simulink model "bus_as_currsource_charging_discharging_final_rearranged"  (R2023a)
settings: Solver=VariableStepAuto  StartTime=0.0  StopTime=10.0  RelTol=1e-3
libraries: spsParallelRLCBranchLib x72, spsCurrentMeasurementLib x27, spsVoltageMeasurementLib x27, spspowerguiLib x25, spsControlledVoltageSourceLib x24, spsVariableResistorLib x24, spsSeriesRLCBranchLib x6, spsMosfetLib x2, sdolib x1, spsControlledCurrentSourceLib x1, spsGroundLib x1
(part 2 of 4)

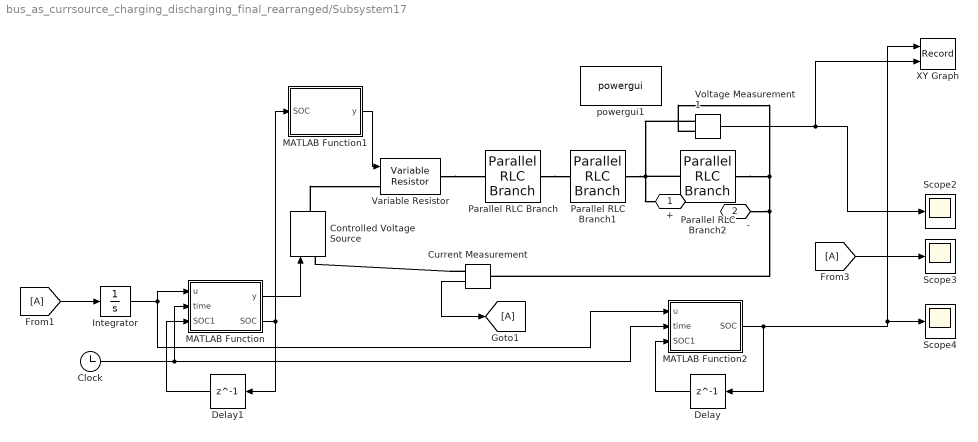
== system bus_as_currsource_charging_discharging_final_rearranged/Subsystem17 ==
  Clock : Clock
  Controlled Voltage Source : spsControlledVoltageSourceLib/Controlled Voltage Source  Initialize=on  Source_Type=DC  Amplitude=0  Phase=0  Frequency=0  Measurements=None
  Current Measurement : spsCurrentMeasurementLib/Current Measurement  PhasorSimulation=off  OutputType=Complex  PSBequivalent=0
  Delay : Delay  DelayLength=1  InitialCondition=0
  Delay1 : Delay  DelayLength=1  InitialCondition=0
  From1 : From
  From3 : From
  Goto1 : Goto
  Integrator : Integrator
  MATLAB Function : MATLAB Function  TreatAsAtomicUnit=on
  MATLAB Function1 : MATLAB Function  TreatAsAtomicUnit=on
  MATLAB Function2 : MATLAB Function  TreatAsAtomicUnit=on
  Parallel RLC Branch : spsParallelRLCBranchLib/Parallel RLC Branch  LConnTagsString=a  RConnTagsString=__new0  BranchType=RC  Resistance=15.5e-3  Inductance=1e-3  SetiL0=off  InitialCurrent=0  Capacitance=1028.7  Setx0=off  InitialVoltage=0  Measurements=None
  Parallel RLC Branch1 : spsParallelRLCBranchLib/Parallel RLC Branch  LConnTagsString=a  RConnTagsString=__new0  BranchType=RC  Resistance=18.3e-3  Inductance=1e-3  SetiL0=off  InitialCurrent=0  Capacitance=5756.6  Setx0=off  InitialVoltage=0  Measurements=None
  Parallel RLC Branch2 : spsParallelRLCBranchLib/Parallel RLC Branch  LConnTagsString=a  RConnTagsString=__new0  BranchType=R  Resistance=1e9  Inductance=1e-3  SetiL0=off  InitialCurrent=0  Capacitance=5756.6  Setx0=off  InitialVoltage=0  Measurements=None
  Scope2 : Scope
  Scope3 : Scope
  Scope4 : Scope
  Variable Resistor : spsVariableResistorLib/Variable Resistor  Rabsmin=1e-3
      settings: LibrarySourceBlock=sps_lib/Passives/Variable Resistor
  Voltage Measurement1 : spsVoltageMeasurementLib/Voltage Measurement  PhasorSimulation=off  OutputType=Complex  PSBequivalent=0
  XY Graph : Record  FileSettingsInternal="{\"entries\":[{\"content\":{\"excelSettings\":{\"content\":{},\"type\":\"Streamout.ExcelSettings\"}},\"type\":\"Streamout.FileSettingStorage\",\"uuid\":\"ba5f6825-ae84-49c8-9f06-d48f38ab3e7c\"}],\"packageUris\":[\"http://schema.mathworks.com/mf0/streamout_blocks/R2020a\"],\"version\":\"1.0\"}"  Layout=[1 1]  SignalsInternal="{\"entries\":[{\"content\":{\"signals\":[{\"content\":{\"blockPath\":[\"untitled/Subsystem17/XY Graph\"],\"dimensions\":[1],\"domain\":\"untitled/Subsystem17/XY Graph\",\"lineColor\":\"#ff6929\",\"port\":1,\"signalID\":782,\"signalName\":\"MATLAB Function2\"},\"type\":\"RecordBlkView.Signal\",\"uuid\":\"a10a1c50-d255-4169-acf7-794a73575721\"},{\"content\":{\"blockPath\":[\"untitled/Subsystem17/XY Graph\"],\"dimensions\":[1],\"domain\":\"untitled/Subsystem17/XY Graph\",\"lineColor\":\"#b746ff\",\"port\":2,\"signalID\":785,\"signalName\":\"Voltage Measurement1\"},\"type\":\"RecordBlkView.Signal\",\"uuid\":\"1a7b2192-97ab-4747-8306-6a319dd4fa57\"}]},\"type\":\"RecordBlkView.InputSignals\",\"uuid\":\"436618d9-ba51-4f23-94da-7eccc7c92e1d\"}],\"packageUris\":[\"http://schema.mathworks.com/mf0/streamout_blocks/R2020a\"],\"version\":\"1.0\"}"  VisualizationBindings="{\"xyplotplugin\":{\"info\":[{\"series\":[],\"subplotID\":1}]}}"  CompatibilityTag=XY
  powergui1 : spspowerguiLib/powergui  Priority=1  SimulationMode=Discrete  SampleTime=2e-7  frequency=60  Iterations=50  frequencyindice=0  Pbase=100e6  ErrMax=1e-4  UnitsV=kV  UnitsW=MW  buscounter=0  FunctionMessages=off  echomessages=off  EnableUseOfTLC=off  CurrentSourceSwitches=off  DisableSnubberDevices=off  DisableRonSwitches=off  DisableVfSwitches=off  DisplayEquations=off  AutomaticDiscreteSolvers=off  SolverType=Tustin/Backward Euler (TBE)  Interpol=off  ExternalGateDelay=off  methode=off  Ts=100  x0status=blocks  SPID=on  SwTol=0  HookPort=off  NonlinearTolerance=1e-4  nMaxIteration=100  ContinueOnMaxIteration=off  RestoreLinks=warning  ResistiveCurrentMeasurement=off  Frange=[0:2:500]  Ylog=off  Xlog=on  ShowGrid=off  save=off  variable=ZData  structure=0  ZoomFFT=off  StartTime=0.0  cycles=1  DisplayStyle=1  fundamental=60  FreqAxis=off  MaxFrequency=1000  frequencyindicesteady=1  RmsSteady=1  display=off
  + : PMIOPort  Side=Right
  - : PMIOPort  Port=2  Side=Left
  wires:
  Current Measurement/1 -> Goto1/1
  From3/1 -> Scope3/1
  Voltage Measurement1/1 -> XY Graph/2, Scope2/1
  MATLAB Function2/1(SOC) -> Delay/1, XY Graph/1, Scope4/1
  From1/1 -> Integrator/1
  MATLAB Function/1(y) -> Controlled Voltage Source/1
  MATLAB Function1/1(y) -> Variable Resistor/1
  Integrator/1 -> MATLAB Function2/1(u), MATLAB Function/1(u)
  Clock/1 -> MATLAB Function2/2(time), MATLAB Function/2(time)
  MATLAB Function/2(SOC) -> Delay1/1, MATLAB Function1/1(SOC)
  Delay/1 -> MATLAB Function2/3(SOC1)
  Delay1/1 -> MATLAB Function/3(SOC1)
  connections:
  Variable Resistor/RConn1 -- Parallel RLC Branch/LConn1
  Parallel RLC Branch1/RConn1 -- Parallel RLC Branch2/LConn1 -- +/RConn1 -- Voltage Measurement1/LConn1
  Voltage Measurement1/LConn2 -- Parallel RLC Branch2/RConn1 -- -/RConn1 -- Current Measurement/LConn1
  Controlled Voltage Source/RConn1 -- Variable Resistor/LConn1
  Current Measurement/RConn1 -- Controlled Voltage Source/LConn1
  Parallel RLC Branch/RConn1 -- Parallel RLC Branch1/LConn1

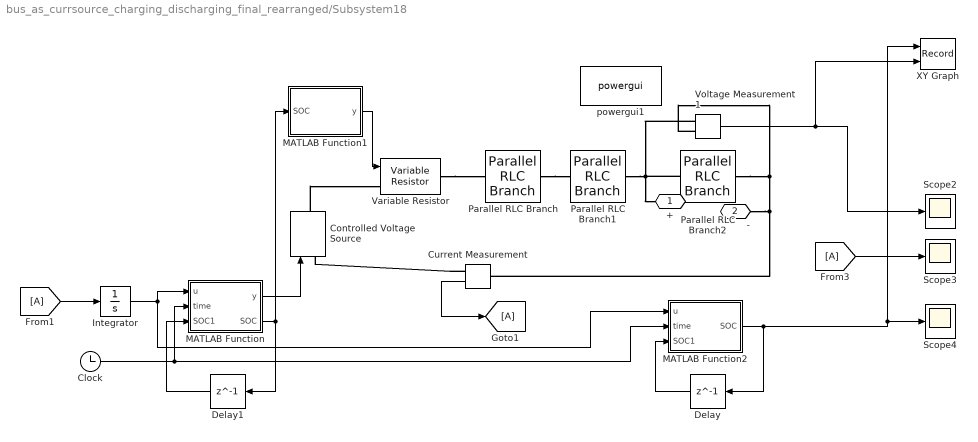
== system bus_as_currsource_charging_discharging_final_rearranged/Subsystem18 ==
  Clock : Clock
  Controlled Voltage Source : spsControlledVoltageSourceLib/Controlled Voltage Source  Initialize=on  Source_Type=DC  Amplitude=0  Phase=0  Frequency=0  Measurements=None
  Current Measurement : spsCurrentMeasurementLib/Current Measurement  PhasorSimulation=off  OutputType=Complex  PSBequivalent=0
  Delay : Delay  DelayLength=1  InitialCondition=0
  Delay1 : Delay  DelayLength=1  InitialCondition=0
  From1 : From
  From3 : From
  Goto1 : Goto
  Integrator : Integrator
  MATLAB Function : MATLAB Function  TreatAsAtomicUnit=on
  MATLAB Function1 : MATLAB Function  TreatAsAtomicUnit=on
  MATLAB Function2 : MATLAB Function  TreatAsAtomicUnit=on
  Parallel RLC Branch : spsParallelRLCBranchLib/Parallel RLC Branch  LConnTagsString=a  RConnTagsString=__new0  BranchType=RC  Resistance=15.5e-3  Inductance=1e-3  SetiL0=off  InitialCurrent=0  Capacitance=1028.7  Setx0=off  InitialVoltage=0  Measurements=None
  Parallel RLC Branch1 : spsParallelRLCBranchLib/Parallel RLC Branch  LConnTagsString=a  RConnTagsString=__new0  BranchType=RC  Resistance=18.3e-3  Inductance=1e-3  SetiL0=off  InitialCurrent=0  Capacitance=5756.6  Setx0=off  InitialVoltage=0  Measurements=None
  Parallel RLC Branch2 : spsParallelRLCBranchLib/Parallel RLC Branch  LConnTagsString=a  RConnTagsString=__new0  BranchType=R  Resistance=1e9  Inductance=1e-3  SetiL0=off  InitialCurrent=0  Capacitance=5756.6  Setx0=off  InitialVoltage=0  Measurements=None
  Scope2 : Scope
  Scope3 : Scope
  Scope4 : Scope
  Variable Resistor : spsVariableResistorLib/Variable Resistor  Rabsmin=1e-3
      settings: LibrarySourceBlock=sps_lib/Passives/Variable Resistor
  Voltage Measurement1 : spsVoltageMeasurementLib/Voltage Measurement  PhasorSimulation=off  OutputType=Complex  PSBequivalent=0
  XY Graph : Record  FileSettingsInternal="{\"entries\":[{\"content\":{\"excelSettings\":{\"content\":{},\"type\":\"Streamout.ExcelSettings\"}},\"type\":\"Streamout.FileSettingStorage\",\"uuid\":\"904955a5-0c01-49ed-b26f-b95637efeaf3\"}],\"packageUris\":[\"http://schema.mathworks.com/mf0/streamout_blocks/R2020a\"],\"version\":\"1.0\"}"  Layout=[1 1]  SignalsInternal="{\"entries\":[{\"content\":{\"signals\":[{\"content\":{\"blockPath\":[\"untitled/Subsystem18/XY Graph\"],\"dimensions\":[1],\"domain\":\"untitled/Subsystem18/XY Graph\",\"lineColor\":\"#64d413\",\"port\":1,\"signalID\":790,\"signalName\":\"MATLAB Function2\"},\"type\":\"RecordBlkView.Signal\",\"uuid\":\"1fb2fe81-24a5-4ae9-8bb1-12b55be0d8f0\"},{\"content\":{\"blockPath\":[\"untitled/Subsystem18/XY Graph\"],\"dimensions\":[1],\"domain\":\"untitled/Subsystem18/XY Graph\",\"lineColor\":\"#ff13a6\",\"port\":2,\"signalID\":793,\"signalName\":\"Voltage Measurement1\"},\"type\":\"RecordBlkView.Signal\",\"uuid\":\"c3accbba-7a16-4831-baea-974c7269be9e\"}]},\"type\":\"RecordBlkView.InputSignals\",\"uuid\":\"9612f47e-78d6-4563-83f2-d5ca8ddd9aa3\"}],\"packageUris\":[\"http://schema.mathworks.com/mf0/streamout_blocks/R2020a\"],\"version\":\"1.0\"}"  VisualizationBindings="{\"xyplotplugin\":{\"info\":[{\"series\":[],\"subplotID\":1}]}}"  CompatibilityTag=XY
  powergui1 : spspowerguiLib/powergui  Priority=1  SimulationMode=Discrete  SampleTime=2e-7  frequency=60  Iterations=50  frequencyindice=0  Pbase=100e6  ErrMax=1e-4  UnitsV=kV  UnitsW=MW  buscounter=0  FunctionMessages=off  echomessages=off  EnableUseOfTLC=off  CurrentSourceSwitches=off  DisableSnubberDevices=off  DisableRonSwitches=off  DisableVfSwitches=off  DisplayEquations=off  AutomaticDiscreteSolvers=off  SolverType=Tustin/Backward Euler (TBE)  Interpol=off  ExternalGateDelay=off  methode=off  Ts=100  x0status=blocks  SPID=on  SwTol=0  HookPort=off  NonlinearTolerance=1e-4  nMaxIteration=100  ContinueOnMaxIteration=off  RestoreLinks=warning  ResistiveCurrentMeasurement=off  Frange=[0:2:500]  Ylog=off  Xlog=on  ShowGrid=off  save=off  variable=ZData  structure=0  ZoomFFT=off  StartTime=0.0  cycles=1  DisplayStyle=1  fundamental=60  FreqAxis=off  MaxFrequency=1000  frequencyindicesteady=1  RmsSteady=1  display=off
  + : PMIOPort  Side=Right
  - : PMIOPort  Port=2  Side=Left
  wires:
  Current Measurement/1 -> Goto1/1
  From3/1 -> Scope3/1
  Voltage Measurement1/1 -> XY Graph/2, Scope2/1
  MATLAB Function2/1(SOC) -> Delay/1, XY Graph/1, Scope4/1
  From1/1 -> Integrator/1
  MATLAB Function/1(y) -> Controlled Voltage Source/1
  MATLAB Function1/1(y) -> Variable Resistor/1
  Integrator/1 -> MATLAB Function2/1(u), MATLAB Function/1(u)
  Clock/1 -> MATLAB Function2/2(time), MATLAB Function/2(time)
  MATLAB Function/2(SOC) -> Delay1/1, MATLAB Function1/1(SOC)
  Delay/1 -> MATLAB Function2/3(SOC1)
  Delay1/1 -> MATLAB Function/3(SOC1)
  connections:
  Variable Resistor/RConn1 -- Parallel RLC Branch/LConn1
  Parallel RLC Branch1/RConn1 -- Parallel RLC Branch2/LConn1 -- +/RConn1 -- Voltage Measurement1/LConn1
  Voltage Measurement1/LConn2 -- Parallel RLC Branch2/RConn1 -- -/RConn1 -- Current Measurement/LConn1
  Controlled Voltage Source/RConn1 -- Variable Resistor/LConn1
  Current Measurement/RConn1 -- Controlled Voltage Source/LConn1
  Parallel RLC Branch/RConn1 -- Parallel RLC Branch1/LConn1

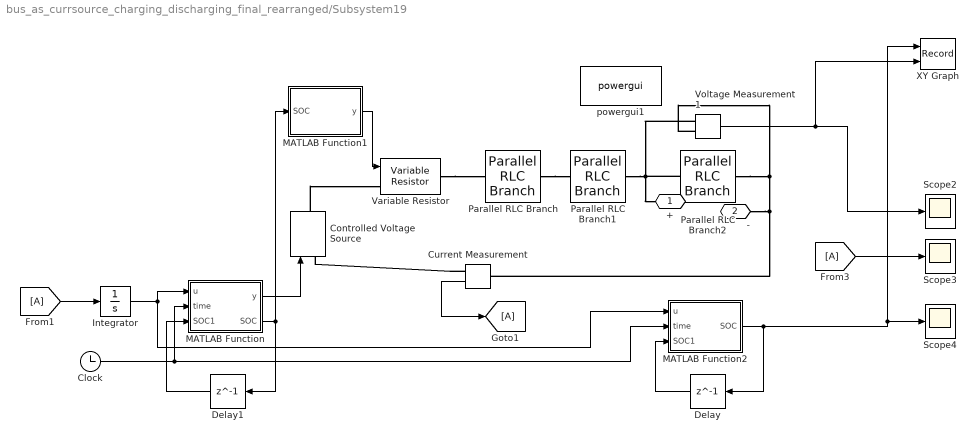
== system bus_as_currsource_charging_discharging_final_rearranged/Subsystem19 ==
  Clock : Clock
  Controlled Voltage Source : spsControlledVoltageSourceLib/Controlled Voltage Source  Initialize=on  Source_Type=DC  Amplitude=0  Phase=0  Frequency=0  Measurements=None
  Current Measurement : spsCurrentMeasurementLib/Current Measurement  PhasorSimulation=off  OutputType=Complex  PSBequivalent=0
  Delay : Delay  DelayLength=1  InitialCondition=0
  Delay1 : Delay  DelayLength=1  InitialCondition=0
  From1 : From
  From3 : From
  Goto1 : Goto
  Integrator : Integrator
  MATLAB Function : MATLAB Function  TreatAsAtomicUnit=on
  MATLAB Function1 : MATLAB Function  TreatAsAtomicUnit=on
  MATLAB Function2 : MATLAB Function  TreatAsAtomicUnit=on
  Parallel RLC Branch : spsParallelRLCBranchLib/Parallel RLC Branch  LConnTagsString=a  RConnTagsString=__new0  BranchType=RC  Resistance=15.5e-3  Inductance=1e-3  SetiL0=off  InitialCurrent=0  Capacitance=1028.7  Setx0=off  InitialVoltage=0  Measurements=None
  Parallel RLC Branch1 : spsParallelRLCBranchLib/Parallel RLC Branch  LConnTagsString=a  RConnTagsString=__new0  BranchType=RC  Resistance=18.3e-3  Inductance=1e-3  SetiL0=off  InitialCurrent=0  Capacitance=5756.6  Setx0=off  InitialVoltage=0  Measurements=None
  Parallel RLC Branch2 : spsParallelRLCBranchLib/Parallel RLC Branch  LConnTagsString=a  RConnTagsString=__new0  BranchType=R  Resistance=1e9  Inductance=1e-3  SetiL0=off  InitialCurrent=0  Capacitance=5756.6  Setx0=off  InitialVoltage=0  Measurements=None
  Scope2 : Scope
  Scope3 : Scope
  Scope4 : Scope
  Variable Resistor : spsVariableResistorLib/Variable Resistor  Rabsmin=1e-3
      settings: LibrarySourceBlock=sps_lib/Passives/Variable Resistor
  Voltage Measurement1 : spsVoltageMeasurementLib/Voltage Measurement  PhasorSimulation=off  OutputType=Complex  PSBequivalent=0
  XY Graph : Record  FileSettingsInternal="{\"entries\":[{\"content\":{\"excelSettings\":{\"content\":{},\"type\":\"Streamout.ExcelSettings\"}},\"type\":\"Streamout.FileSettingStorage\",\"uuid\":\"49e6397f-4cd4-4408-b704-a90deb42e929\"}],\"packageUris\":[\"http://schema.mathworks.com/mf0/streamout_blocks/R2020a\"],\"version\":\"1.0\"}"  Layout=[1 1]  SignalsInternal="{\"entries\":[{\"content\":{\"signals\":[{\"content\":{\"blockPath\":[\"untitled/Subsystem19/XY Graph\"],\"dimensions\":[1],\"domain\":\"untitled/Subsystem19/XY Graph\",\"lineColor\":\"#fe330a\",\"port\":1,\"signalID\":798,\"signalName\":\"MATLAB Function2\"},\"type\":\"RecordBlkView.Signal\",\"uuid\":\"20b7caa4-e151-45a3-bb88-2e4765233750\"},{\"content\":{\"blockPath\":[\"untitled/Subsystem19/XY Graph\"],\"dimensions\":[1],\"domain\":\"untitled/Subsystem19/XY Graph\",\"lineColor\":\"#22b573\",\"port\":2,\"signalID\":801,\"signalName\":\"Voltage Measurement1\"},\"type\":\"RecordBlkView.Signal\",\"uuid\":\"9713df5b-9710-418f-a0db-9a9919584767\"}]},\"type\":\"RecordBlkView.InputSignals\",\"uuid\":\"2c966842-6eda-4904-b11c-392011e40ac1\"}],\"packageUris\":[\"http://schema.mathworks.com/mf0/streamout_blocks/R2020a\"],\"version\":\"1.0\"}"  VisualizationBindings="{\"xyplotplugin\":{\"info\":[{\"series\":[],\"subplotID\":1}]}}"  CompatibilityTag=XY
  powergui1 : spspowerguiLib/powergui  Priority=1  SimulationMode=Discrete  SampleTime=2e-7  frequency=60  Iterations=50  frequencyindice=0  Pbase=100e6  ErrMax=1e-4  UnitsV=kV  UnitsW=MW  buscounter=0  FunctionMessages=off  echomessages=off  EnableUseOfTLC=off  CurrentSourceSwitches=off  DisableSnubberDevices=off  DisableRonSwitches=off  DisableVfSwitches=off  DisplayEquations=off  AutomaticDiscreteSolvers=off  SolverType=Tustin/Backward Euler (TBE)  Interpol=off  ExternalGateDelay=off  methode=off  Ts=100  x0status=blocks  SPID=on  SwTol=0  HookPort=off  NonlinearTolerance=1e-4  nMaxIteration=100  ContinueOnMaxIteration=off  RestoreLinks=warning  ResistiveCurrentMeasurement=off  Frange=[0:2:500]  Ylog=off  Xlog=on  ShowGrid=off  save=off  variable=ZData  structure=0  ZoomFFT=off  StartTime=0.0  cycles=1  DisplayStyle=1  fundamental=60  FreqAxis=off  MaxFrequency=1000  frequencyindicesteady=1  RmsSteady=1  display=off
  + : PMIOPort  Side=Right
  - : PMIOPort  Port=2  Side=Left
  wires:
  Current Measurement/1 -> Goto1/1
  From3/1 -> Scope3/1
  Voltage Measurement1/1 -> XY Graph/2, Scope2/1
  MATLAB Function2/1(SOC) -> Delay/1, XY Graph/1, Scope4/1
  From1/1 -> Integrator/1
  MATLAB Function/1(y) -> Controlled Voltage Source/1
  MATLAB Function1/1(y) -> Variable Resistor/1
  Integrator/1 -> MATLAB Function2/1(u), MATLAB Function/1(u)
  Clock/1 -> MATLAB Function2/2(time), MATLAB Function/2(time)
  MATLAB Function/2(SOC) -> Delay1/1, MATLAB Function1/1(SOC)
  Delay/1 -> MATLAB Function2/3(SOC1)
  Delay1/1 -> MATLAB Function/3(SOC1)
  connections:
  Variable Resistor/RConn1 -- Parallel RLC Branch/LConn1
  Parallel RLC Branch1/RConn1 -- Parallel RLC Branch2/LConn1 -- +/RConn1 -- Voltage Measurement1/LConn1
  Voltage Measurement1/LConn2 -- Parallel RLC Branch2/RConn1 -- -/RConn1 -- Current Measurement/LConn1
  Controlled Voltage Source/RConn1 -- Variable Resistor/LConn1
  Current Measurement/RConn1 -- Controlled Voltage Source/LConn1
  Parallel RLC Branch/RConn1 -- Parallel RLC Branch1/LConn1

== system bus_as_currsource_charging_discharging_final_rearranged/Subsystem2 ==
  Clock : Clock
  Controlled Voltage Source : spsControlledVoltageSourceLib/Controlled Voltage Source  Initialize=on  Source_Type=DC  Amplitude=0  Phase=0  Frequency=0  Measurements=None
  Current Measurement : spsCurrentMeasurementLib/Current Measurement  PhasorSimulation=off  OutputType=Complex  PSBequivalent=0
  Delay : Delay  DelayLength=1  InitialCondition=0
  Delay1 : Delay  DelayLength=1  InitialCondition=0
  From1 : From
  From3 : From
  Goto1 : Goto
  Integrator : Integrator
  MATLAB Function : MATLAB Function  TreatAsAtomicUnit=on
  MATLAB Function1 : MATLAB Function  TreatAsAtomicUnit=on
  MATLAB Function2 : MATLAB Function  TreatAsAtomicUnit=on
  Parallel RLC Branch : spsParallelRLCBranchLib/Parallel RLC Branch  LConnTagsString=a  RConnTagsString=__new0  BranchType=RC  Resistance=15.5e-3  Inductance=1e-3  SetiL0=off  InitialCurrent=0  Capacitance=1028.7  Setx0=off  InitialVoltage=0  Measurements=None
  Parallel RLC Branch1 : spsParallelRLCBranchLib/Parallel RLC Branch  LConnTagsString=a  RConnTagsString=__new0  BranchType=RC  Resistance=18.3e-3  Inductance=1e-3  SetiL0=off  InitialCurrent=0  Capacitance=5756.6  Setx0=off  InitialVoltage=0  Measurements=None
  Parallel RLC Branch2 : spsParallelRLCBranchLib/Parallel RLC Branch  LConnTagsString=a  RConnTagsString=__new0  BranchType=R  Resistance=1e9  Inductance=1e-3  SetiL0=off  InitialCurrent=0  Capacitance=5756.6  Setx0=off  InitialVoltage=0  Measurements=None
  Scope2 : Scope
  Scope3 : Scope
  Scope4 : Scope
  Variable Resistor : spsVariableResistorLib/Variable Resistor  Rabsmin=1e-3
      settings: LibrarySourceBlock=sps_lib/Passives/Variable Resistor
  Voltage Measurement1 : spsVoltageMeasurementLib/Voltage Measurement  PhasorSimulation=off  OutputType=Complex  PSBequivalent=0
  XY Graph : Record  FileSettingsInternal="{\"entries\":[{\"content\":{\"excelSettings\":{\"content\":{},\"type\":\"Streamout.ExcelSettings\"}},\"type\":\"Streamout.FileSettingStorage\",\"uuid\":\"e662f745-69cc-49f8-b12c-20846ce44359\"}],\"packageUris\":[\"http://schema.mathworks.com/mf0/streamout_blocks/R2020a\"],\"version\":\"1.0\"}"  Layout=[1 1]  SignalsInternal="{\"entries\":[{\"content\":{\"signals\":[{\"content\":{\"blockPath\":[\"untitled/Subsystem2/XY Graph\"],\"dimensions\":[1],\"domain\":\"untitled/Subsystem2/XY Graph\",\"lineColor\":\"#0072bd\",\"port\":1,\"signalID\":806,\"signalName\":\"MATLAB Function2\"},\"type\":\"RecordBlkView.Signal\",\"uuid\":\"74a79339-a0a1-47aa-ad7f-e0a02e4a4241\"},{\"content\":{\"blockPath\":[\"untitled/Subsystem2/XY Graph\"],\"dimensions\":[1],\"domain\":\"untitled/Subsystem2/XY Graph\",\"lineColor\":\"#d95319\",\"port\":2,\"signalID\":809,\"signalName\":\"Voltage Measurement1\"},\"type\":\"RecordBlkView.Signal\",\"uuid\":\"59fded46-9d8b-4ac5-9d49-55c2866e06d0\"}]},\"type\":\"RecordBlkView.InputSignals\",\"uuid\":\"0a2f4e3d-6747-49af-9ef6-e89a65c13c10\"}],\"packageUris\":[\"http://schema.mathworks.com/mf0/streamout_blocks/R2020a\"],\"version\":\"1.0\"}"  VisualizationBindings="{\"xyplotplugin\":{\"info\":[{\"series\":[],\"subplotID\":1}]}}"  CompatibilityTag=XY
  powergui1 : spspowerguiLib/powergui  Priority=1  SimulationMode=Discrete  SampleTime=2e-7  frequency=60  Iterations=50  frequencyindice=0  Pbase=100e6  ErrMax=1e-4  UnitsV=kV  UnitsW=MW  buscounter=0  FunctionMessages=off  echomessages=off  EnableUseOfTLC=off  CurrentSourceSwitches=off  DisableSnubberDevices=off  DisableRonSwitches=off  DisableVfSwitches=off  DisplayEquations=off  AutomaticDiscreteSolvers=off  SolverType=Tustin/Backward Euler (TBE)  Interpol=off  ExternalGateDelay=off  methode=off  Ts=100  x0status=blocks  SPID=on  SwTol=0  HookPort=off  NonlinearTolerance=1e-4  nMaxIteration=100  ContinueOnMaxIteration=off  RestoreLinks=warning  ResistiveCurrentMeasurement=off  Frange=[0:2:500]  Ylog=off  Xlog=on  ShowGrid=off  save=off  variable=ZData  structure=0  ZoomFFT=off  StartTime=0.0  cycles=1  DisplayStyle=1  fundamental=60  FreqAxis=off  MaxFrequency=1000  frequencyindicesteady=1  RmsSteady=1  display=off
  + : PMIOPort  Side=Right
  - : PMIOPort  Port=2  Side=Left
  wires:
  Current Measurement/1 -> Goto1/1
  From3/1 -> Scope3/1
  Voltage Measurement1/1 -> XY Graph/2, Scope2/1
  MATLAB Function2/1(SOC) -> Delay/1, XY Graph/1, Scope4/1
  From1/1 -> Integrator/1
  MATLAB Function/1(y) -> Controlled Voltage Source/1
  MATLAB Function1/1(y) -> Variable Resistor/1
  Integrator/1 -> MATLAB Function2/1(u), MATLAB Function/1(u)
  Clock/1 -> MATLAB Function2/2(time), MATLAB Function/2(time)
  MATLAB Function/2(SOC) -> Delay1/1, MATLAB Function1/1(SOC)
  Delay/1 -> MATLAB Function2/3(SOC1)
  Delay1/1 -> MATLAB Function/3(SOC1)
  connections:
  Variable Resistor/RConn1 -- Parallel RLC Branch/LConn1
  Parallel RLC Branch1/RConn1 -- Parallel RLC Branch2/LConn1 -- +/RConn1 -- Voltage Measurement1/LConn1
  Voltage Measurement1/LConn2 -- Parallel RLC Branch2/RConn1 -- -/RConn1 -- Current Measurement/LConn1
  Controlled Voltage Source/RConn1 -- Variable Resistor/LConn1
  Current Measurement/RConn1 -- Controlled Voltage Source/LConn1
  Parallel RLC Branch/RConn1 -- Parallel RLC Branch1/LConn1

== system bus_as_currsource_charging_discharging_final_rearranged/Subsystem20 ==
  Clock : Clock
  Controlled Voltage Source : spsControlledVoltageSourceLib/Controlled Voltage Source  Initialize=on  Source_Type=DC  Amplitude=0  Phase=0  Frequency=0  Measurements=None
  Current Measurement : spsCurrentMeasurementLib/Current Measurement  PhasorSimulation=off  OutputType=Complex  PSBequivalent=0
  Delay : Delay  DelayLength=1  InitialCondition=0
  Delay1 : Delay  DelayLength=1  InitialCondition=0
  From1 : From
  From3 : From
  Goto1 : Goto
  Integrator : Integrator
  MATLAB Function : MATLAB Function  TreatAsAtomicUnit=on
  MATLAB Function1 : MATLAB Function  TreatAsAtomicUnit=on
  MATLAB Function2 : MATLAB Function  TreatAsAtomicUnit=on
  Parallel RLC Branch : spsParallelRLCBranchLib/Parallel RLC Branch  LConnTagsString=a  RConnTagsString=__new0  BranchType=RC  Resistance=15.5e-3  Inductance=1e-3  SetiL0=off  InitialCurrent=0  Capacitance=1028.7  Setx0=off  InitialVoltage=0  Measurements=None
  Parallel RLC Branch1 : spsParallelRLCBranchLib/Parallel RLC Branch  LConnTagsString=a  RConnTagsString=__new0  BranchType=RC  Resistance=18.3e-3  Inductance=1e-3  SetiL0=off  InitialCurrent=0  Capacitance=5756.6  Setx0=off  InitialVoltage=0  Measurements=None
  Parallel RLC Branch2 : spsParallelRLCBranchLib/Parallel RLC Branch  LConnTagsString=a  RConnTagsString=__new0  BranchType=R  Resistance=1e9  Inductance=1e-3  SetiL0=off  InitialCurrent=0  Capacitance=5756.6  Setx0=off  InitialVoltage=0  Measurements=None
  Scope2 : Scope
  Scope3 : Scope
  Scope4 : Scope
  Variable Resistor : spsVariableResistorLib/Variable Resistor  Rabsmin=1e-3
      settings: LibrarySourceBlock=sps_lib/Passives/Variable Resistor
  Voltage Measurement1 : spsVoltageMeasurementLib/Voltage Measurement  PhasorSimulation=off  OutputType=Complex  PSBequivalent=0
  XY Graph : Record  FileSettingsInternal="{\"entries\":[{\"content\":{\"excelSettings\":{\"content\":{},\"type\":\"Streamout.ExcelSettings\"}},\"type\":\"Streamout.FileSettingStorage\",\"uuid\":\"b9cd57a9-9675-4bd3-81a7-674b40545c75\"}],\"packageUris\":[\"http://schema.mathworks.com/mf0/streamout_blocks/R2020a\"],\"version\":\"1.0\"}"  Layout=[1 1]  SignalsInternal="{\"entries\":[{\"content\":{\"signals\":[{\"content\":{\"blockPath\":[\"untitled/Subsystem20/XY Graph\"],\"dimensions\":[1],\"domain\":\"untitled/Subsystem20/XY Graph\",\"lineColor\":\"#edb120\",\"port\":1,\"signalID\":814,\"signalName\":\"MATLAB Function2\"},\"type\":\"RecordBlkView.Signal\",\"uuid\":\"d625c523-3804-4fa7-bc4a-cd5d4b0b6e39\"},{\"content\":{\"blockPath\":[\"untitled/Subsystem20/XY Graph\"],\"dimensions\":[1],\"domain\":\"untitled/Subsystem20/XY Graph\",\"lineColor\":\"#7e2f8e\",\"port\":2,\"signalID\":817,\"signalName\":\"Voltage Measurement1\"},\"type\":\"RecordBlkView.Signal\",\"uuid\":\"d19b35e0-7b80-4888-a05f-93661bf810a0\"}]},\"type\":\"RecordBlkView.InputSignals\",\"uuid\":\"6bb0314d-672c-4472-be59-eec52ca77f93\"}],\"packageUris\":[\"http://schema.mathworks.com/mf0/streamout_blocks/R2020a\"],\"version\":\"1.0\"}"  VisualizationBindings="{\"xyplotplugin\":{\"info\":[{\"series\":[],\"subplotID\":1}]}}"  CompatibilityTag=XY
  powergui1 : spspowerguiLib/powergui  Priority=1  SimulationMode=Discrete  SampleTime=2e-7  frequency=60  Iterations=50  frequencyindice=0  Pbase=100e6  ErrMax=1e-4  UnitsV=kV  UnitsW=MW  buscounter=0  FunctionMessages=off  echomessages=off  EnableUseOfTLC=off  CurrentSourceSwitches=off  DisableSnubberDevices=off  DisableRonSwitches=off  DisableVfSwitches=off  DisplayEquations=off  AutomaticDiscreteSolvers=off  SolverType=Tustin/Backward Euler (TBE)  Interpol=off  ExternalGateDelay=off  methode=off  Ts=100  x0status=blocks  SPID=on  SwTol=0  HookPort=off  NonlinearTolerance=1e-4  nMaxIteration=100  ContinueOnMaxIteration=off  RestoreLinks=warning  ResistiveCurrentMeasurement=off  Frange=[0:2:500]  Ylog=off  Xlog=on  ShowGrid=off  save=off  variable=ZData  structure=0  ZoomFFT=off  StartTime=0.0  cycles=1  DisplayStyle=1  fundamental=60  FreqAxis=off  MaxFrequency=1000  frequencyindicesteady=1  RmsSteady=1  display=off
  + : PMIOPort  Side=Right
  - : PMIOPort  Port=2  Side=Left
  wires:
  Current Measurement/1 -> Goto1/1
  From3/1 -> Scope3/1
  Voltage Measurement1/1 -> XY Graph/2, Scope2/1
  MATLAB Function2/1(SOC) -> Delay/1, XY Graph/1, Scope4/1
  From1/1 -> Integrator/1
  MATLAB Function/1(y) -> Controlled Voltage Source/1
  MATLAB Function1/1(y) -> Variable Resistor/1
  Integrator/1 -> MATLAB Function2/1(u), MATLAB Function/1(u)
  Clock/1 -> MATLAB Function2/2(time), MATLAB Function/2(time)
  MATLAB Function/2(SOC) -> Delay1/1, MATLAB Function1/1(SOC)
  Delay/1 -> MATLAB Function2/3(SOC1)
  Delay1/1 -> MATLAB Function/3(SOC1)
  connections:
  Variable Resistor/RConn1 -- Parallel RLC Branch/LConn1
  Parallel RLC Branch1/RConn1 -- Parallel RLC Branch2/LConn1 -- +/RConn1 -- Voltage Measurement1/LConn1
  Voltage Measurement1/LConn2 -- Parallel RLC Branch2/RConn1 -- -/RConn1 -- Current Measurement/LConn1
  Controlled Voltage Source/RConn1 -- Variable Resistor/LConn1
  Current Measurement/RConn1 -- Controlled Voltage Source/LConn1
  Parallel RLC Branch/RConn1 -- Parallel RLC Branch1/LConn1

== system bus_as_currsource_charging_discharging_final_rearranged/Subsystem21 ==
  Clock : Clock
  Controlled Voltage Source : spsControlledVoltageSourceLib/Controlled Voltage Source  Initialize=on  Source_Type=DC  Amplitude=0  Phase=0  Frequency=0  Measurements=None
  Current Measurement : spsCurrentMeasurementLib/Current Measurement  PhasorSimulation=off  OutputType=Complex  PSBequivalent=0
  Delay : Delay  DelayLength=1  InitialCondition=0
  Delay1 : Delay  DelayLength=1  InitialCondition=0
  From1 : From
  From3 : From
  Goto1 : Goto
  Integrator : Integrator
  MATLAB Function : MATLAB Function  TreatAsAtomicUnit=on
  MATLAB Function1 : MATLAB Function  TreatAsAtomicUnit=on
  MATLAB Function2 : MATLAB Function  TreatAsAtomicUnit=on
  Parallel RLC Branch : spsParallelRLCBranchLib/Parallel RLC Branch  LConnTagsString=a  RConnTagsString=__new0  BranchType=RC  Resistance=15.5e-3  Inductance=1e-3  SetiL0=off  InitialCurrent=0  Capacitance=1028.7  Setx0=off  InitialVoltage=0  Measurements=None
  Parallel RLC Branch1 : spsParallelRLCBranchLib/Parallel RLC Branch  LConnTagsString=a  RConnTagsString=__new0  BranchType=RC  Resistance=18.3e-3  Inductance=1e-3  SetiL0=off  InitialCurrent=0  Capacitance=5756.6  Setx0=off  InitialVoltage=0  Measurements=None
  Parallel RLC Branch2 : spsParallelRLCBranchLib/Parallel RLC Branch  LConnTagsString=a  RConnTagsString=__new0  BranchType=R  Resistance=1e9  Inductance=1e-3  SetiL0=off  InitialCurrent=0  Capacitance=5756.6  Setx0=off  InitialVoltage=0  Measurements=None
  Scope2 : Scope
  Scope3 : Scope
  Scope4 : Scope
  Variable Resistor : spsVariableResistorLib/Variable Resistor  Rabsmin=1e-3
      settings: LibrarySourceBlock=sps_lib/Passives/Variable Resistor
  Voltage Measurement1 : spsVoltageMeasurementLib/Voltage Measurement  PhasorSimulation=off  OutputType=Complex  PSBequivalent=0
  XY Graph : Record  FileSettingsInternal="{\"entries\":[{\"content\":{\"excelSettings\":{\"content\":{},\"type\":\"Streamout.ExcelSettings\"}},\"type\":\"Streamout.FileSettingStorage\",\"uuid\":\"2aa9a4d4-1198-43c9-b6a5-531cb0b57d60\"}],\"packageUris\":[\"http://schema.mathworks.com/mf0/streamout_blocks/R2020a\"],\"version\":\"1.0\"}"  Layout=[1 1]  SignalsInternal="{\"entries\":[{\"content\":{\"signals\":[{\"content\":{\"blockPath\":[\"untitled/Subsystem21/XY Graph\"],\"dimensions\":[1],\"domain\":\"untitled/Subsystem21/XY Graph\",\"lineColor\":\"#77ac30\",\"port\":1,\"signalID\":822,\"signalName\":\"MATLAB Function2\"},\"type\":\"RecordBlkView.Signal\",\"uuid\":\"0d291af4-fe64-4eb4-8c95-ecd6ca26bd6a\"},{\"content\":{\"blockPath\":[\"untitled/Subsystem21/XY Graph\"],\"dimensions\":[1],\"domain\":\"untitled/Subsystem21/XY Graph\",\"lineColor\":\"#4dbeee\",\"port\":2,\"signalID\":825,\"signalName\":\"Voltage Measurement1\"},\"type\":\"RecordBlkView.Signal\",\"uuid\":\"561a3197-f113-47c4-b4d1-2a6a4a0e839d\"}]},\"type\":\"RecordBlkView.InputSignals\",\"uuid\":\"ec12e811-28df-4e1b-b5ba-617bc867fb63\"}],\"packageUris\":[\"http://schema.mathworks.com/mf0/streamout_blocks/R2020a\"],\"version\":\"1.0\"}"  VisualizationBindings="{\"xyplotplugin\":{\"info\":[{\"series\":[],\"subplotID\":1}]}}"  CompatibilityTag=XY
  powergui1 : spspowerguiLib/powergui  Priority=1  SimulationMode=Discrete  SampleTime=2e-7  frequency=60  Iterations=50  frequencyindice=0  Pbase=100e6  ErrMax=1e-4  UnitsV=kV  UnitsW=MW  buscounter=0  FunctionMessages=off  echomessages=off  EnableUseOfTLC=off  CurrentSourceSwitches=off  DisableSnubberDevices=off  DisableRonSwitches=off  DisableVfSwitches=off  DisplayEquations=off  AutomaticDiscreteSolvers=off  SolverType=Tustin/Backward Euler (TBE)  Interpol=off  ExternalGateDelay=off  methode=off  Ts=100  x0status=blocks  SPID=on  SwTol=0  HookPort=off  NonlinearTolerance=1e-4  nMaxIteration=100  ContinueOnMaxIteration=off  RestoreLinks=warning  ResistiveCurrentMeasurement=off  Frange=[0:2:500]  Ylog=off  Xlog=on  ShowGrid=off  save=off  variable=ZData  structure=0  ZoomFFT=off  StartTime=0.0  cycles=1  DisplayStyle=1  fundamental=60  FreqAxis=off  MaxFrequency=1000  frequencyindicesteady=1  RmsSteady=1  display=off
  + : PMIOPort  Side=Right
  - : PMIOPort  Port=2  Side=Left
  wires:
  Current Measurement/1 -> Goto1/1
  From3/1 -> Scope3/1
  Voltage Measurement1/1 -> XY Graph/2, Scope2/1
  MATLAB Function2/1(SOC) -> Delay/1, XY Graph/1, Scope4/1
  From1/1 -> Integrator/1
  MATLAB Function/1(y) -> Controlled Voltage Source/1
  MATLAB Function1/1(y) -> Variable Resistor/1
  Integrator/1 -> MATLAB Function2/1(u), MATLAB Function/1(u)
  Clock/1 -> MATLAB Function2/2(time), MATLAB Function/2(time)
  MATLAB Function/2(SOC) -> Delay1/1, MATLAB Function1/1(SOC)
  Delay/1 -> MATLAB Function2/3(SOC1)
  Delay1/1 -> MATLAB Function/3(SOC1)
  connections:
  Variable Resistor/RConn1 -- Parallel RLC Branch/LConn1
  Parallel RLC Branch1/RConn1 -- Parallel RLC Branch2/LConn1 -- +/RConn1 -- Voltage Measurement1/LConn1
  Voltage Measurement1/LConn2 -- Parallel RLC Branch2/RConn1 -- -/RConn1 -- Current Measurement/LConn1
  Controlled Voltage Source/RConn1 -- Variable Resistor/LConn1
  Current Measurement/RConn1 -- Controlled Voltage Source/LConn1
  Parallel RLC Branch/RConn1 -- Parallel RLC Branch1/LConn1

== system bus_as_currsource_charging_discharging_final_rearranged/Subsystem22 ==
  Clock : Clock
  Controlled Voltage Source : spsControlledVoltageSourceLib/Controlled Voltage Source  Initialize=on  Source_Type=DC  Amplitude=0  Phase=0  Frequency=0  Measurements=None
  Current Measurement : spsCurrentMeasurementLib/Current Measurement  PhasorSimulation=off  OutputType=Complex  PSBequivalent=0
  Delay : Delay  DelayLength=1  InitialCondition=0
  Delay1 : Delay  DelayLength=1  InitialCondition=0
  From1 : From
  From3 : From
  Goto1 : Goto
  Integrator : Integrator
  MATLAB Function : MATLAB Function  TreatAsAtomicUnit=on
  MATLAB Function1 : MATLAB Function  TreatAsAtomicUnit=on
  MATLAB Function2 : MATLAB Function  TreatAsAtomicUnit=on
  Parallel RLC Branch : spsParallelRLCBranchLib/Parallel RLC Branch  LConnTagsString=a  RConnTagsString=__new0  BranchType=RC  Resistance=15.5e-3  Inductance=1e-3  SetiL0=off  InitialCurrent=0  Capacitance=1028.7  Setx0=off  InitialVoltage=0  Measurements=None
  Parallel RLC Branch1 : spsParallelRLCBranchLib/Parallel RLC Branch  LConnTagsString=a  RConnTagsString=__new0  BranchType=RC  Resistance=18.3e-3  Inductance=1e-3  SetiL0=off  InitialCurrent=0  Capacitance=5756.6  Setx0=off  InitialVoltage=0  Measurements=None
  Parallel RLC Branch2 : spsParallelRLCBranchLib/Parallel RLC Branch  LConnTagsString=a  RConnTagsString=__new0  BranchType=R  Resistance=1e9  Inductance=1e-3  SetiL0=off  InitialCurrent=0  Capacitance=5756.6  Setx0=off  InitialVoltage=0  Measurements=None
  Scope2 : Scope
  Scope3 : Scope
  Scope4 : Scope
  Variable Resistor : spsVariableResistorLib/Variable Resistor  Rabsmin=1e-3
      settings: LibrarySourceBlock=sps_lib/Passives/Variable Resistor
  Voltage Measurement1 : spsVoltageMeasurementLib/Voltage Measurement  PhasorSimulation=off  OutputType=Complex  PSBequivalent=0
  XY Graph : Record  FileSettingsInternal="{\"entries\":[{\"content\":{\"excelSettings\":{\"content\":{},\"type\":\"Streamout.ExcelSettings\"}},\"type\":\"Streamout.FileSettingStorage\",\"uuid\":\"11f2ab75-dc85-4da5-b0b4-c1e5270eac03\"}],\"packageUris\":[\"http://schema.mathworks.com/mf0/streamout_blocks/R2020a\"],\"version\":\"1.0\"}"  Layout=[1 1]  SignalsInternal="{\"entries\":[{\"content\":{\"signals\":[{\"content\":{\"blockPath\":[\"untitled/Subsystem22/XY Graph\"],\"dimensions\":[1],\"domain\":\"untitled/Subsystem22/XY Graph\",\"lineColor\":\"#a2142f\",\"port\":1,\"signalID\":830,\"signalName\":\"MATLAB Function2\"},\"type\":\"RecordBlkView.Signal\",\"uuid\":\"9a886c97-4532-4703-a17f-b540e6f40f77\"},{\"content\":{\"blockPath\":[\"untitled/Subsystem22/XY Graph\"],\"dimensions\":[1],\"domain\":\"untitled/Subsystem22/XY Graph\",\"lineColor\":\"#139fff\",\"port\":2,\"signalID\":833,\"signalName\":\"Voltage Measurement1\"},\"type\":\"RecordBlkView.Signal\",\"uuid\":\"ba7a69d0-8a5d-49b1-aa1d-c7084a12b5e8\"}]},\"type\":\"RecordBlkView.InputSignals\",\"uuid\":\"a5c2090a-4c0a-4b0c-a0ef-ad6ffeb6fa96\"}],\"packageUris\":[\"http://schema.mathworks.com/mf0/streamout_blocks/R2020a\"],\"version\":\"1.0\"}"  VisualizationBindings="{\"xyplotplugin\":{\"info\":[{\"series\":[],\"subplotID\":1}]}}"  CompatibilityTag=XY
  powergui1 : spspowerguiLib/powergui  Priority=1  SimulationMode=Discrete  SampleTime=2e-7  frequency=60  Iterations=50  frequencyindice=0  Pbase=100e6  ErrMax=1e-4  UnitsV=kV  UnitsW=MW  buscounter=0  FunctionMessages=off  echomessages=off  EnableUseOfTLC=off  CurrentSourceSwitches=off  DisableSnubberDevices=off  DisableRonSwitches=off  DisableVfSwitches=off  DisplayEquations=off  AutomaticDiscreteSolvers=off  SolverType=Tustin/Backward Euler (TBE)  Interpol=off  ExternalGateDelay=off  methode=off  Ts=100  x0status=blocks  SPID=on  SwTol=0  HookPort=off  NonlinearTolerance=1e-4  nMaxIteration=100  ContinueOnMaxIteration=off  RestoreLinks=warning  ResistiveCurrentMeasurement=off  Frange=[0:2:500]  Ylog=off  Xlog=on  ShowGrid=off  save=off  variable=ZData  structure=0  ZoomFFT=off  StartTime=0.0  cycles=1  DisplayStyle=1  fundamental=60  FreqAxis=off  MaxFrequency=1000  frequencyindicesteady=1  RmsSteady=1  display=off
  + : PMIOPort  Side=Right
  - : PMIOPort  Port=2  Side=Left
  wires:
  Current Measurement/1 -> Goto1/1
  From3/1 -> Scope3/1
  Voltage Measurement1/1 -> XY Graph/2, Scope2/1
  MATLAB Function2/1(SOC) -> Delay/1, XY Graph/1, Scope4/1
  From1/1 -> Integrator/1
  MATLAB Function/1(y) -> Controlled Voltage Source/1
  MATLAB Function1/1(y) -> Variable Resistor/1
  Integrator/1 -> MATLAB Function2/1(u), MATLAB Function/1(u)
  Clock/1 -> MATLAB Function2/2(time), MATLAB Function/2(time)
  MATLAB Function/2(SOC) -> Delay1/1, MATLAB Function1/1(SOC)
  Delay/1 -> MATLAB Function2/3(SOC1)
  Delay1/1 -> MATLAB Function/3(SOC1)
  connections:
  Variable Resistor/RConn1 -- Parallel RLC Branch/LConn1
  Parallel RLC Branch1/RConn1 -- Parallel RLC Branch2/LConn1 -- +/RConn1 -- Voltage Measurement1/LConn1
  Voltage Measurement1/LConn2 -- Parallel RLC Branch2/RConn1 -- -/RConn1 -- Current Measurement/LConn1
  Controlled Voltage Source/RConn1 -- Variable Resistor/LConn1
  Current Measurement/RConn1 -- Controlled Voltage Source/LConn1
  Parallel RLC Branch/RConn1 -- Parallel RLC Branch1/LConn1

== system bus_as_currsource_charging_discharging_final_rearranged/Subsystem23 ==
  Clock : Clock
  Controlled Voltage Source : spsControlledVoltageSourceLib/Controlled Voltage Source  Initialize=on  Source_Type=DC  Amplitude=0  Phase=0  Frequency=0  Measurements=None
  Current Measurement : spsCurrentMeasurementLib/Current Measurement  PhasorSimulation=off  OutputType=Complex  PSBequivalent=0
  Delay : Delay  DelayLength=1  InitialCondition=0
  Delay1 : Delay  DelayLength=1  InitialCondition=0
  From1 : From
  From3 : From
  Goto1 : Goto
  Integrator : Integrator
  MATLAB Function : MATLAB Function  TreatAsAtomicUnit=on
  MATLAB Function1 : MATLAB Function  TreatAsAtomicUnit=on
  MATLAB Function2 : MATLAB Function  TreatAsAtomicUnit=on
  Parallel RLC Branch : spsParallelRLCBranchLib/Parallel RLC Branch  LConnTagsString=a  RConnTagsString=__new0  BranchType=RC  Resistance=15.5e-3  Inductance=1e-3  SetiL0=off  InitialCurrent=0  Capacitance=1028.7  Setx0=off  InitialVoltage=0  Measurements=None
  Parallel RLC Branch1 : spsParallelRLCBranchLib/Parallel RLC Branch  LConnTagsString=a  RConnTagsString=__new0  BranchType=RC  Resistance=18.3e-3  Inductance=1e-3  SetiL0=off  InitialCurrent=0  Capacitance=5756.6  Setx0=off  InitialVoltage=0  Measurements=None
  Parallel RLC Branch2 : spsParallelRLCBranchLib/Parallel RLC Branch  LConnTagsString=a  RConnTagsString=__new0  BranchType=R  Resistance=1e9  Inductance=1e-3  SetiL0=off  InitialCurrent=0  Capacitance=5756.6  Setx0=off  InitialVoltage=0  Measurements=None
  Scope2 : Scope
  Scope3 : Scope
  Scope4 : Scope
  Variable Resistor : spsVariableResistorLib/Variable Resistor  Rabsmin=1e-3
      settings: LibrarySourceBlock=sps_lib/Passives/Variable Resistor
  Voltage Measurement1 : spsVoltageMeasurementLib/Voltage Measurement  PhasorSimulation=off  OutputType=Complex  PSBequivalent=0
  XY Graph : Record  FileSettingsInternal="{\"entries\":[{\"content\":{\"excelSettings\":{\"content\":{},\"type\":\"Streamout.ExcelSettings\"}},\"type\":\"Streamout.FileSettingStorage\",\"uuid\":\"4507d666-d6cd-4b94-9588-b6f195b9fedb\"}],\"packageUris\":[\"http://schema.mathworks.com/mf0/streamout_blocks/R2020a\"],\"version\":\"1.0\"}"  Layout=[1 1]  SignalsInternal="{\"entries\":[{\"content\":{\"signals\":[{\"content\":{\"blockPath\":[\"untitled/Subsystem23/XY Graph\"],\"dimensions\":[1],\"domain\":\"untitled/Subsystem23/XY Graph\",\"lineColor\":\"#ff6929\",\"port\":1,\"signalID\":838,\"signalName\":\"MATLAB Function2\"},\"type\":\"RecordBlkView.Signal\",\"uuid\":\"f4d36bbb-bacb-4cfd-960d-7f6fe2510a89\"},{\"content\":{\"blockPath\":[\"untitled/Subsystem23/XY Graph\"],\"dimensions\":[1],\"domain\":\"untitled/Subsystem23/XY Graph\",\"lineColor\":\"#b746ff\",\"port\":2,\"signalID\":841,\"signalName\":\"Voltage Measurement1\"},\"type\":\"RecordBlkView.Signal\",\"uuid\":\"d517bb7c-6bc7-48ba-8e0f-83d7f4d5133a\"}]},\"type\":\"RecordBlkView.InputSignals\",\"uuid\":\"6cc68769-996e-4abe-900c-2cee26e138db\"}],\"packageUris\":[\"http://schema.mathworks.com/mf0/streamout_blocks/R2020a\"],\"version\":\"1.0\"}"  VisualizationBindings="{\"xyplotplugin\":{\"info\":[{\"series\":[],\"subplotID\":1}]}}"  CompatibilityTag=XY
  powergui1 : spspowerguiLib/powergui  Priority=1  SimulationMode=Discrete  SampleTime=2e-7  frequency=60  Iterations=50  frequencyindice=0  Pbase=100e6  ErrMax=1e-4  UnitsV=kV  UnitsW=MW  buscounter=0  FunctionMessages=off  echomessages=off  EnableUseOfTLC=off  CurrentSourceSwitches=off  DisableSnubberDevices=off  DisableRonSwitches=off  DisableVfSwitches=off  DisplayEquations=off  AutomaticDiscreteSolvers=off  SolverType=Tustin/Backward Euler (TBE)  Interpol=off  ExternalGateDelay=off  methode=off  Ts=100  x0status=blocks  SPID=on  SwTol=0  HookPort=off  NonlinearTolerance=1e-4  nMaxIteration=100  ContinueOnMaxIteration=off  RestoreLinks=warning  ResistiveCurrentMeasurement=off  Frange=[0:2:500]  Ylog=off  Xlog=on  ShowGrid=off  save=off  variable=ZData  structure=0  ZoomFFT=off  StartTime=0.0  cycles=1  DisplayStyle=1  fundamental=60  FreqAxis=off  MaxFrequency=1000  frequencyindicesteady=1  RmsSteady=1  display=off
  + : PMIOPort  Side=Right
  - : PMIOPort  Port=2  Side=Left
  wires:
  Current Measurement/1 -> Goto1/1
  From3/1 -> Scope3/1
  Voltage Measurement1/1 -> XY Graph/2, Scope2/1
  MATLAB Function2/1(SOC) -> Delay/1, XY Graph/1, Scope4/1
  From1/1 -> Integrator/1
  MATLAB Function/1(y) -> Controlled Voltage Source/1
  MATLAB Function1/1(y) -> Variable Resistor/1
  Integrator/1 -> MATLAB Function2/1(u), MATLAB Function/1(u)
  Clock/1 -> MATLAB Function2/2(time), MATLAB Function/2(time)
  MATLAB Function/2(SOC) -> Delay1/1, MATLAB Function1/1(SOC)
  Delay/1 -> MATLAB Function2/3(SOC1)
  Delay1/1 -> MATLAB Function/3(SOC1)
  connections:
  Variable Resistor/RConn1 -- Parallel RLC Branch/LConn1
  Parallel RLC Branch1/RConn1 -- Parallel RLC Branch2/LConn1 -- +/RConn1 -- Voltage Measurement1/LConn1
  Voltage Measurement1/LConn2 -- Parallel RLC Branch2/RConn1 -- -/RConn1 -- Current Measurement/LConn1
  Controlled Voltage Source/RConn1 -- Variable Resistor/LConn1
  Current Measurement/RConn1 -- Controlled Voltage Source/LConn1
  Parallel RLC Branch/RConn1 -- Parallel RLC Branch1/LConn1

== system bus_as_currsource_charging_discharging_final_rearranged/Subsystem24 ==
  Clock : Clock
  Controlled Voltage Source : spsControlledVoltageSourceLib/Controlled Voltage Source  Initialize=on  Source_Type=DC  Amplitude=0  Phase=0  Frequency=0  Measurements=None
  Current Measurement : spsCurrentMeasurementLib/Current Measurement  PhasorSimulation=off  OutputType=Complex  PSBequivalent=0
  Delay : Delay  DelayLength=1  InitialCondition=0
  Delay1 : Delay  DelayLength=1  InitialCondition=0
  From1 : From
  From3 : From
  Goto1 : Goto
  Integrator : Integrator
  MATLAB Function : MATLAB Function  TreatAsAtomicUnit=on
  MATLAB Function1 : MATLAB Function  TreatAsAtomicUnit=on
  MATLAB Function2 : MATLAB Function  TreatAsAtomicUnit=on
  Parallel RLC Branch : spsParallelRLCBranchLib/Parallel RLC Branch  LConnTagsString=a  RConnTagsString=__new0  BranchType=RC  Resistance=15.5e-3  Inductance=1e-3  SetiL0=off  InitialCurrent=0  Capacitance=1028.7  Setx0=off  InitialVoltage=0  Measurements=None
  Parallel RLC Branch1 : spsParallelRLCBranchLib/Parallel RLC Branch  LConnTagsString=a  RConnTagsString=__new0  BranchType=RC  Resistance=18.3e-3  Inductance=1e-3  SetiL0=off  InitialCurrent=0  Capacitance=5756.6  Setx0=off  InitialVoltage=0  Measurements=None
  Parallel RLC Branch2 : spsParallelRLCBranchLib/Parallel RLC Branch  LConnTagsString=a  RConnTagsString=__new0  BranchType=R  Resistance=1e9  Inductance=1e-3  SetiL0=off  InitialCurrent=0  Capacitance=5756.6  Setx0=off  InitialVoltage=0  Measurements=None
  Scope2 : Scope
  Scope3 : Scope
  Scope4 : Scope
  Variable Resistor : spsVariableResistorLib/Variable Resistor  Rabsmin=1e-3
      settings: LibrarySourceBlock=sps_lib/Passives/Variable Resistor
  Voltage Measurement1 : spsVoltageMeasurementLib/Voltage Measurement  PhasorSimulation=off  OutputType=Complex  PSBequivalent=0
  XY Graph : Record  FileSettingsInternal="{\"entries\":[{\"content\":{\"excelSettings\":{\"content\":{},\"type\":\"Streamout.ExcelSettings\"}},\"type\":\"Streamout.FileSettingStorage\",\"uuid\":\"6d097b1f-e2ef-4430-a153-1310af4205e5\"}],\"packageUris\":[\"http://schema.mathworks.com/mf0/streamout_blocks/R2020a\"],\"version\":\"1.0\"}"  Layout=[1 1]  SignalsInternal="{\"entries\":[{\"content\":{\"signals\":[{\"content\":{\"blockPath\":[\"untitled/Subsystem24/XY Graph\"],\"dimensions\":[1],\"domain\":\"untitled/Subsystem24/XY Graph\",\"lineColor\":\"#64d413\",\"port\":1,\"signalID\":846,\"signalName\":\"MATLAB Function2\"},\"type\":\"RecordBlkView.Signal\",\"uuid\":\"e7622e7e-bffb-4900-9ef5-2399709765c0\"},{\"content\":{\"blockPath\":[\"untitled/Subsystem24/XY Graph\"],\"dimensions\":[1],\"domain\":\"untitled/Subsystem24/XY Graph\",\"lineColor\":\"#ff13a6\",\"port\":2,\"signalID\":849,\"signalName\":\"Voltage Measurement1\"},\"type\":\"RecordBlkView.Signal\",\"uuid\":\"246d3dc2-6613-4a8e-9434-fed76b26703c\"}]},\"type\":\"RecordBlkView.InputSignals\",\"uuid\":\"2ea0af46-97d9-45f5-9b01-07a0eff2bf4d\"}],\"packageUris\":[\"http://schema.mathworks.com/mf0/streamout_blocks/R2020a\"],\"version\":\"1.0\"}"  VisualizationBindings="{\"xyplotplugin\":{\"info\":[{\"series\":[],\"subplotID\":1}]}}"  CompatibilityTag=XY
  powergui1 : spspowerguiLib/powergui  Priority=1  SimulationMode=Discrete  SampleTime=2e-7  frequency=60  Iterations=50  frequencyindice=0  Pbase=100e6  ErrMax=1e-4  UnitsV=kV  UnitsW=MW  buscounter=0  FunctionMessages=off  echomessages=off  EnableUseOfTLC=off  CurrentSourceSwitches=off  DisableSnubberDevices=off  DisableRonSwitches=off  DisableVfSwitches=off  DisplayEquations=off  AutomaticDiscreteSolvers=off  SolverType=Tustin/Backward Euler (TBE)  Interpol=off  ExternalGateDelay=off  methode=off  Ts=100  x0status=blocks  SPID=on  SwTol=0  HookPort=off  NonlinearTolerance=1e-4  nMaxIteration=100  ContinueOnMaxIteration=off  RestoreLinks=warning  ResistiveCurrentMeasurement=off  Frange=[0:2:500]  Ylog=off  Xlog=on  ShowGrid=off  save=off  variable=ZData  structure=0  ZoomFFT=off  StartTime=0.0  cycles=1  DisplayStyle=1  fundamental=60  FreqAxis=off  MaxFrequency=1000  frequencyindicesteady=1  RmsSteady=1  display=off
  + : PMIOPort  Side=Right
  - : PMIOPort  Port=2  Side=Left
  wires:
  Current Measurement/1 -> Goto1/1
  From3/1 -> Scope3/1
  Voltage Measurement1/1 -> XY Graph/2, Scope2/1
  MATLAB Function2/1(SOC) -> Delay/1, XY Graph/1, Scope4/1
  From1/1 -> Integrator/1
  MATLAB Function/1(y) -> Controlled Voltage Source/1
  MATLAB Function1/1(y) -> Variable Resistor/1
  Integrator/1 -> MATLAB Function2/1(u), MATLAB Function/1(u)
  Clock/1 -> MATLAB Function2/2(time), MATLAB Function/2(time)
  MATLAB Function/2(SOC) -> Delay1/1, MATLAB Function1/1(SOC)
  Delay/1 -> MATLAB Function2/3(SOC1)
  Delay1/1 -> MATLAB Function/3(SOC1)
  connections:
  Variable Resistor/RConn1 -- Parallel RLC Branch/LConn1
  Parallel RLC Branch1/RConn1 -- Parallel RLC Branch2/LConn1 -- +/RConn1 -- Voltage Measurement1/LConn1
  Voltage Measurement1/LConn2 -- Parallel RLC Branch2/RConn1 -- -/RConn1 -- Current Measurement/LConn1
  Controlled Voltage Source/RConn1 -- Variable Resistor/LConn1
  Current Measurement/RConn1 -- Controlled Voltage Source/LConn1
  Parallel RLC Branch/RConn1 -- Parallel RLC Branch1/LConn1
